simulink model "exp4"  (R2024b)
settings: Solver=VariableStepAuto  StartTime=0.0  StopTime=10.0  RelTol=1e-3
libraries: spspowerguiLib x1
settings Model: Creator=shaur  LastModifiedBy=shaur

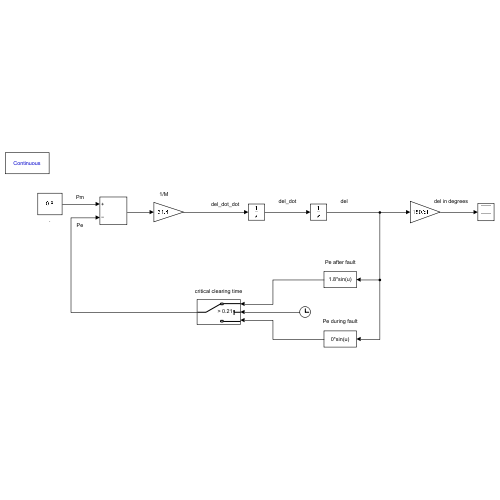
[thumbnail: Simulink's stored preview of the top-level diagram]
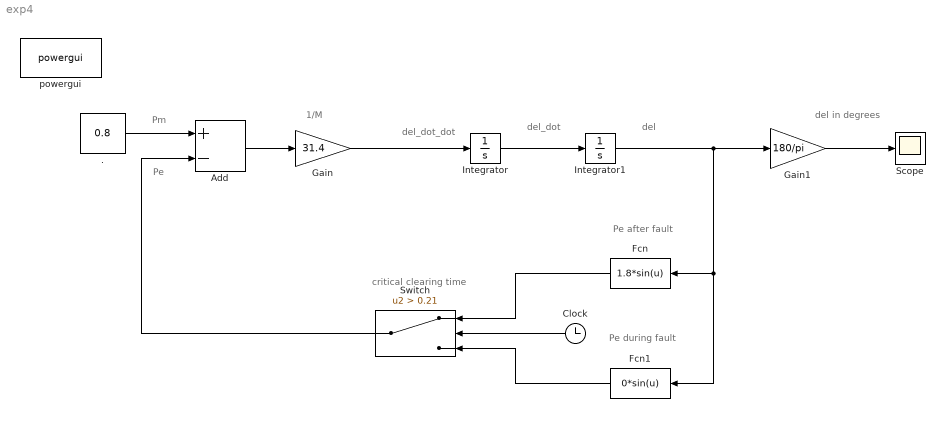
== system exp4 ==
  note: del in degrees
  note: critical clearing time
  note: Pe during fault
  note: Pe after fault
  note: del
  note: del_dot
  note: del_dot_dot
  note: 1/M
  note: Pm
  note: Pe
  . : Constant  Value=0.8
  Add : Sum  Inputs=+-
  Clock : Clock
  Fcn : Fcn  Expr=1.8*sin(u)
  Fcn1 : Fcn  Expr=0*sin(u)
  Gain : Gain  Gain=31.4
  Gain1 : Gain  Gain=180/pi
  Integrator : Integrator
  Integrator1 : Integrator  InitialCondition=0.46
  Scope : Scope
  Switch : Switch  Criteria=u2 > Threshold  Threshold=0.21  SaturateOnIntegerOverflow=off  InputSameDT=off
  powergui : spspowerguiLib/powergui  Priority=1  SimulationMode=Continuous  SampleTime=50e-6  frequency=60  Iterations=50  frequencyindice=60  Pbase=100e6  ErrMax=1e-4  UnitsV=kV  UnitsW=MW  buscounter=0  FunctionMessages=off  echomessages=off  EnableUseOfTLC=off  CurrentSourceSwitches=off  DisableSnubberDevices=off  DisableRonSwitches=off  DisableVfSwitches=off  DisplayEquations=off  AutomaticDiscreteSolvers=off  SolverType=Tustin/Backward Euler (TBE)  Interpol=off  ExternalGateDelay=off  methode=off  Ts=100  x0status=blocks  SPID=on  SwTol=0  HookPort=off  NonlinearTolerance=1e-4  nMaxIteration=100  ContinueOnMaxIteration=off  RestoreLinks=warning  ResistiveCurrentMeasurement=off  Frange=[0:2:500]  Ylog=off  Xlog=on  ShowGrid=off  save=off  variable=ZData  structure=0  ZoomFFT=off  StartTime=0.0  cycles=1  DisplayStyle=1  fundamental=60  FreqAxis=off  MaxFrequency=1000  frequencyindicesteady=1  RmsSteady=1  display=off
  wires:
  ./1 -> Add/1
  Add/1 -> Gain/1
  Gain/1 -> Integrator/1
  Integrator/1 -> Integrator1/1
  Integrator1/1 -> Fcn1/1, Fcn/1, Gain1/1
  Gain1/1 -> Scope/1
  Fcn/1 -> Switch/1
  Clock/1 -> Switch/2
  Fcn1/1 -> Switch/3
  Switch/1 -> Add/2
